simulink model "Laba1"  (R2020a)
settings: Solver=VariableStepAuto  StartTime=0.0  StopTime=10.0  RelTol=1e-3
settings Model: Creator=LinkL  LastModifiedBy=LinkL

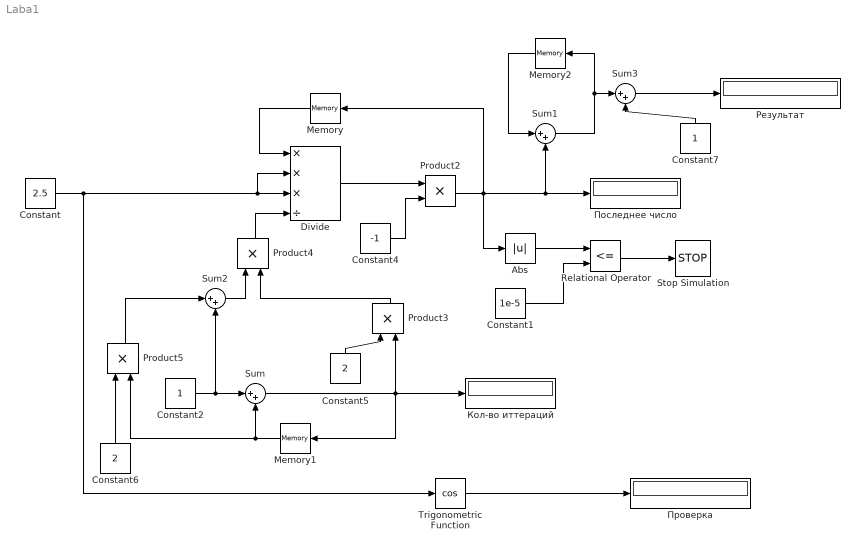
== system Laba1 ==
  Abs : Abs
  Constant : Constant  Value=2.5
  Constant1 : Constant  Value=1e-5
  Constant2 : Constant
  Constant4 : Constant  Value=-1
  Constant5 : Constant  Value=2
  Constant6 : Constant  Value=2
  Constant7 : Constant
  Divide : Product  Inputs=***/
  Memory : Memory  InitialCondition=1
  Memory1 : Memory
  Memory2 : Memory
  Product{2..5} (4 alike) : Product
  Relational Operator : RelationalOperator  Operator=<=  OutDataTypeStr=boolean  RndMeth=Simplest
  Stop Simulation : Stop
  Sum{,1..3} (4 alike) : Sum  Inputs=|++
  Trigonometric Function : Trigonometry  Operator=cos
  Кол-во иттераций : Display
  Последнее число : Display
  Проверка : Display
  Результат : Display
  wires:
  Constant/1 -> Divide/3, Divide/2, Trigonometric Function/1
  Memory/1 -> Divide/1
  Sum/1 -> Memory1/1, Product3/2, Кол-во иттераций/1
  Constant2/1 -> Sum/1, Sum2/2
  Abs/1 -> Relational Operator/1
  Constant1/1 -> Relational Operator/2
  Relational Operator/1 -> Stop Simulation/1
  Memory2/1 -> Sum1/1
  Sum1/1 -> Sum3/1, Memory2/1
  Trigonometric Function/1 -> Проверка/1
  Divide/1 -> Product2/1
  Constant4/1 -> Product2/2
  Product2/1 -> Abs/1, Memory/1, Последнее число/1, Sum1/2
  Memory1/1 -> Product5/2, Sum/2
  Constant5/1 -> Product3/1
  Product4/1 -> Divide/4
  Product3/1 -> Product4/2
  Constant6/1 -> Product5/1
  Sum2/1 -> Product4/1
  Product5/1 -> Sum2/1
  Constant7/1 -> Sum3/2
  Sum3/1 -> Результат/1
